simulink model "qhug_8"  (R2021a)
settings: Solver=ode4  StartTime=0.0  StopTime=500  FixedStep=1  MaxStep=0.1  RelTol=1e-3
settings Model: Creator=daoist  LastModifiedBy=daoist

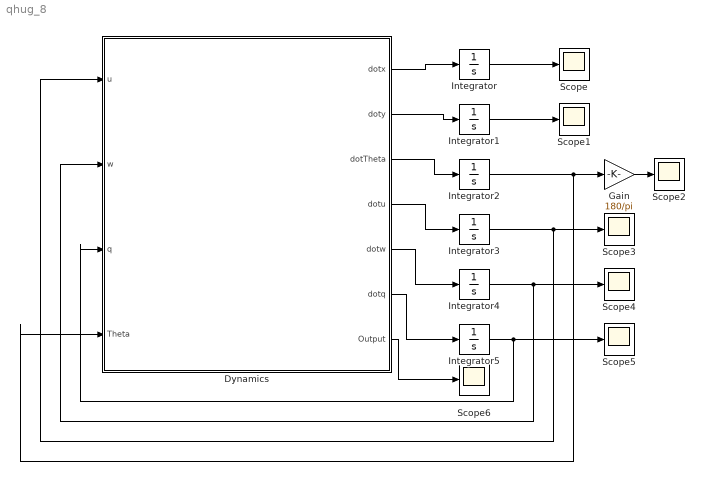
== system qhug_8 ==
  Dynamics : Subsystem
  Gain : Gain  Gain=180/pi
  Integrator{,1..2,4..5} (5 alike) : Integrator
  Integrator3 : Integrator  InitialCondition=0.01
  Scope{,1..6} (7 alike) : Scope
  wires:
  Dynamics/1(dotx) -> Integrator/1
  Dynamics/6(dotq) -> Integrator5/1
  Dynamics/5(dotw) -> Integrator4/1
  Dynamics/4(dotu) -> Integrator3/1
  Dynamics/3(dotTheta) -> Integrator2/1
  Dynamics/2(doty) -> Integrator1/1
  Integrator/1 -> Scope/1
  Integrator1/1 -> Scope1/1
  Integrator2/1 -> Gain/1, Dynamics/4(Theta)
  Integrator3/1 -> Scope3/1, Dynamics/1(u)
  Integrator4/1 -> Scope4/1, Dynamics/2(w)
  Integrator5/1 -> Scope5/1, Dynamics/3(q)
  Gain/1 -> Scope2/1
  Dynamics/7(Output) -> Scope6/1

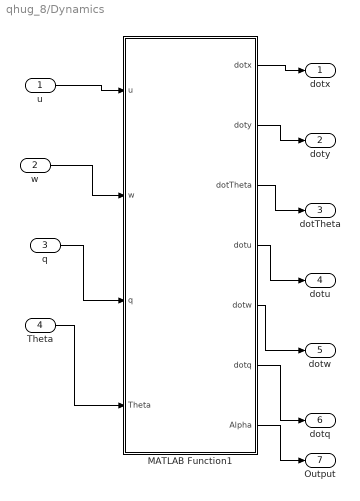
== system qhug_8/Dynamics ==
  u : Inport
  w : Inport  Port=2
  q : Inport  Port=3
  Theta : Inport  Port=4
  MATLAB Function1 : MATLAB Function  TreatAsAtomicUnit=on
  dotx : Outport
  doty : Outport  Port=2
  dotTheta : Outport  Port=3
  dotu : Outport  Port=4
  dotw : Outport  Port=5
  dotq : Outport  Port=6
  Output : Outport  Port=7
  wires:
  MATLAB Function1/1(dotx) -> dotx/1
  MATLAB Function1/2(doty) -> doty/1
  MATLAB Function1/3(dotTheta) -> dotTheta/1
  MATLAB Function1/4(dotu) -> dotu/1
  MATLAB Function1/5(dotw) -> dotw/1
  MATLAB Function1/6(dotq) -> dotq/1
  u/1 -> MATLAB Function1/1(u)
  w/1 -> MATLAB Function1/2(w)
  q/1 -> MATLAB Function1/3(q)
  Theta/1 -> MATLAB Function1/4(Theta)
  MATLAB Function1/7(Alpha) -> Output/1

== matlab function qhug_8/Dynamics/MATLAB Function1 ==
  data: u input; dotx output; w input; q input; Theta input; doty output; dotTheta output; dotu output; dotw output; dotq output; Alpha output
function [dotx, doty, dotTheta, dotu, dotw,dotq, Alpha] = fcn(u, w, q, Theta )
m_b = 0.1668;
r_p1 = 0.019;

m_rb = 53;
m_p = 15;
m_d = 68;
r_b1 = 0.75;
r_p3 = 0.014;
J_f2 = 9.19;
J_rb2 = 15.27;

K_d0 = 9.79;
K_d = 541.01;
K_l0 = 0;
K_l = 622.62;
K_m0 = -1.02;
K_m = -39.53;
K_q = -183.27;
M_f1 = 3.15;
M_f3 = 71.37;

g= 9.81;

V = sqrt(u^2 + w^2);
Alpha = atan(w/u);
D = (K_d0 + K_d * Alpha^2) * V^2;
L = (K_l0 + K_l * Alpha) * V^2;
T_2 = (K_m0 + K_m * Alpha + K_q * q) * V^2';
J_2 = J_rb2 + J_f2;
A = J_2 + m_p * (r_p1^2 + r_p3^2) + m_b * r_b1^2;

m = m_rb + m_p + m_b;
m_0 = m-m_d;


AAA = [ M_f1+m , 0, m_p*r_p3;
    0, M_f3+m, m_p*r_p1+m_b*r_b1;
    m_p*r_p3, -(m_p*r_p1+m_b*r_b1), A;];


B = [-D*cos(Alpha)+L*sin(Alpha)-m_0*g*sin(Theta)-q*w*(M_f3+m)+q^2*(m_p*r_p1+m_b*r_b1),...
    -D*sin(Alpha)-L*cos(Alpha)+m_0*g*sin(Theta)+q*u*(M_f1+m)+q^2*m_p*r_p3,...
    T_2-(m_p*r_p1+m_b*r_b1)*g*cos(Theta)+u*w*(M_f3-M_f1-m_p)-m_p*r_p3*g*sin(Theta)-u*q*m_p*r_p3-u*q*(m_p*r_p1+m_b*r_b1);];

out = inv(AAA) * B';
dotu = out(1);
dotw = out(2);
dotq = out(3);

dotx = u*cos(Theta)+w*sin(Theta);
doty = -u*sin(Theta)+w*cos(Theta);
dotTheta = q;
